simulink model "Ex_7"  (R2020a)
settings: Solver=VariableStepAuto  StartTime=0.0  StopTime=10.0  RelTol=1e-3
values from neighbouring files (symbols this model uses):
  B = 0.0025    [m6.m]    (also in m7.m)
  J = 0.02365    [m6.m]    (also in m7.m)
  La = 0.12    [m6.m]    (also in m7.m)
  Laf = 0.0675    [m7.m]
  Lf = 0.3    [m7.m]
  Ra = 1.50    (= 1.5)    [m6.m]    (also in m7.m)
  Rf = 0.7    [m7.m]
  Va = 240    [m7.m]
settings Model: Creator=abhin  LastModifiedBy=abhin

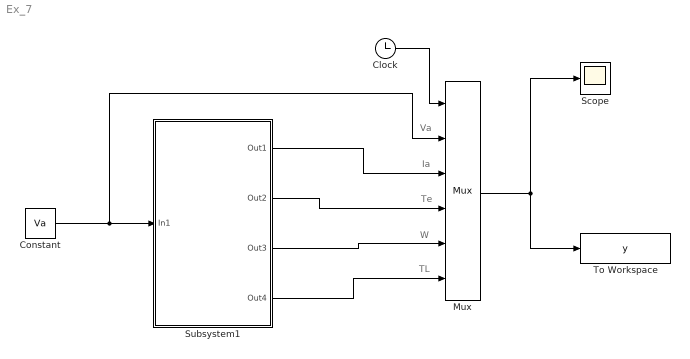
== system Ex_7 ==
  note: Va
  note: TL
  note: W
  note: Te
  note: Ia
  Clock : Clock
  Constant : Constant  Value=Va  SampleTime=1e-3
  Mux : Mux  Inputs=6
  Scope : Scope
  Subsystem1 : Subsystem
  To Workspace : ToWorkspace  VariableName=y  SaveFormat=Structure  SampleTime=-1
      settings: Save2DSignal=2-D array (concatenate along first dimension)
  wires:
  Constant/1 -> Mux/2, Subsystem1/1(In1)
  Clock/1 -> Mux/1
  Mux/1 -> To Workspace/1, Scope/1
  Subsystem1/1(Out1) -> Mux/3
  Subsystem1/2(Out2) -> Mux/4
  Subsystem1/3(Out3) -> Mux/5
  Subsystem1/4(Out4) -> Mux/6

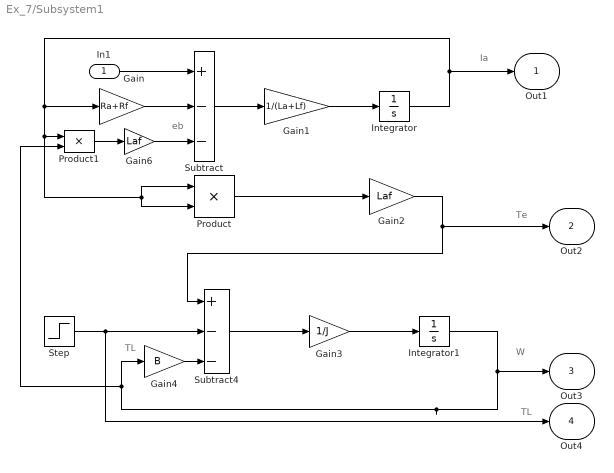
== system Ex_7/Subsystem1 ==
  note: eb
  note: TL
  note: TL
  note: Te
  note: Ia
  note: W
  In1 : Inport
  Gain : Gain  Gain=Ra+Rf
  Gain1 : Gain  Gain=1/(La+Lf)
  Gain2 : Gain  Gain=Laf
  Gain3 : Gain  Gain=1/J
  Gain4 : Gain  Gain=B
  Gain6 : Gain  Gain=Laf
  Integrator : Integrator
  Integrator1 : Integrator
  Product : Product
  Product1 : Product
  Step : Step  Time=3  After=20  SampleTime=0
  Subtract : Sum  Inputs=+--
  Subtract4 : Sum  Inputs=+--
  Out1 : Outport
  Out2 : Outport  Port=2
  Out3 : Outport  Port=3
  Out4 : Outport  Port=4
  wires:
  In1/1 -> Subtract/1
  Gain/1 -> Subtract/2
  Subtract/1 -> Gain1/1
  Gain1/1 -> Integrator/1
  Integrator/1 -> Out1/1, Gain/1, Product1/1, Product/2, Product/1
  Gain2/1 -> Out2/1, Subtract4/1
  Product/1 -> Gain2/1
  Subtract4/1 -> Gain3/1
  Integrator1/1 -> Out3/1, Product1/2, Gain4/1
  Gain3/1 -> Integrator1/1
  Gain4/1 -> Subtract4/3
  Step/1 -> Out4/1, Subtract4/2
  Gain6/1 -> Subtract/3
  Product1/1 -> Gain6/1
